simulink model "Simulasyon"  (R2022b)
settings: Solver=FixedStepDiscrete  StartTime=0.0  StopTime=0.05  FixedStep=1e-7  RelTol=1e-3
undefined symbols (not defined in the file): Ion, Lithium
libraries: spsSeriesRLCBranchLib x10, spsMosfetLib x8, spsPWMGenerator2LevelLib x5, spsThreePhaseVIMeasurementLib x4, spsThreePhaseSeriesRLCBranchLib x4, spsVoltageMeasurementLib x3, spsThreePhaseParallelRLCLoadLib x2, spsDCVoltageSourceLib x2, spsIGBTLib x2, spsThreePhaseBreakerLib x2, spsBatteryLib x1, spsBoostConverterLib x1
settings Model: Creator=ERKAM  LastModifiedBy=ERKAM
settings DataIOCC: ReturnWorkspaceOutputs=off

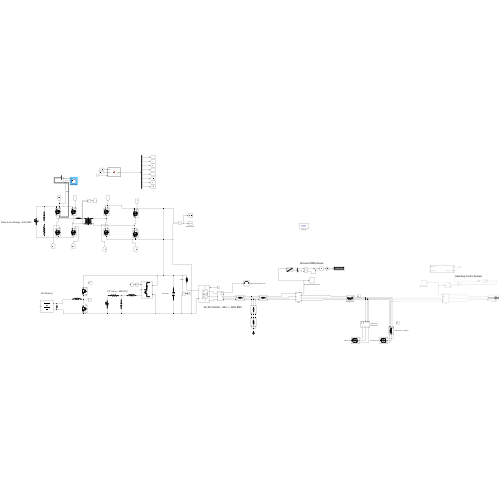
[thumbnail: Simulink's stored preview of the top-level diagram]
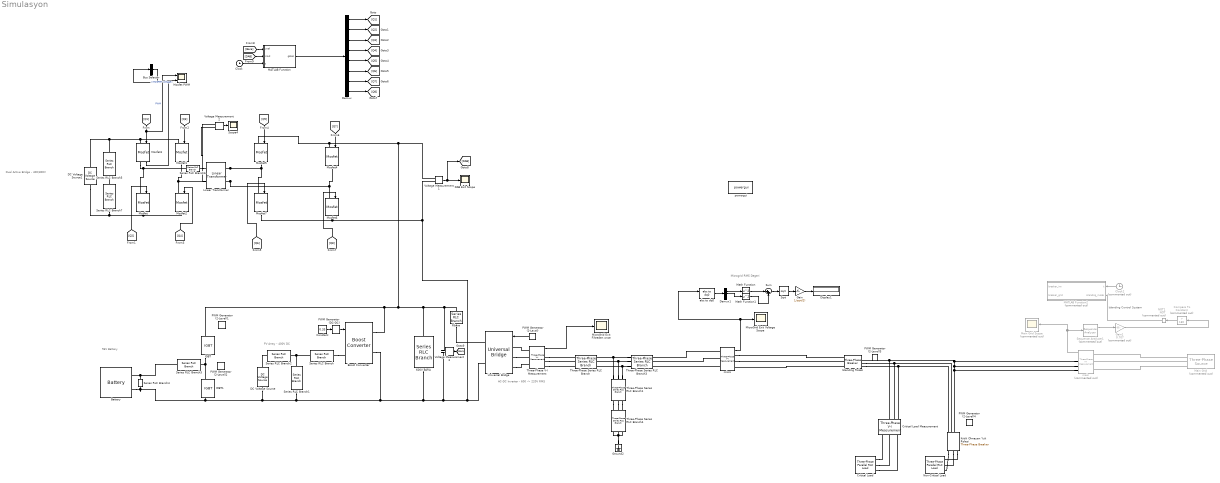
== system Simulasyon ==
  note: Islanding Control System
  note: AC-DC Inverter - 600 -> 220V RMS
  note: Dual Active Bridge - 400/800V
  note: PV Array - 400V DC
  note: 96V Battery
  note: Microgrid RMS Degeri
  600V BARA : spsSeriesRLCBranchLib/Series RLC Branch  LConnTagsString=__new0  RConnTagsString=__new0  BranchType=C  Resistance=1  Inductance=1e-3  SetiL0=off  InitialCurrent=0  Capacitance=100e-6  Setx0=on  InitialVoltage=600  Measurements=None
  Battery : spsBatteryLib/Battery  BatType=Lithium-Ion  ShowTempParam=off  ThermalPreset=no  ShowAgeParam=off  NomV=96  NomQ=100  SOC=100  Batt_Tr=30  PresetModel=on  MaxQ=100  MinV=72  FullV=111.7428  Dis_rate=43.4783  R=0.0096  Normal_OP=90.4348  expZone="[103.717      4.913043]"  current=[6.5 13 32.5]  Units=Time  Tci=20  NomT=20  T2=-30  MaxQ2=4.8  FullV2=7.1  Normal_OP2=5.655  expZone2="[6.58           1]"  Rca=0.6  ti=2000  Dp=0  Neq0=0  Tsim=1e6  Ta1=25  Qeol=5.4*0.9  Reol=0.013333*1.2  Char_age=[2.3478, 3]  Dis_age=[2.3478, 10]  N1=1500  N2=10500  N3=1000  N4=1400  Ta2=45  N5=950
  Boost Converter : spsBoostConverterLib/Boost Converter  ModelType=Switching devices  Ron=1e-3  Rs=1e6  Cs=inf  Vforward=[0,0]  Ron_Diode=1e-3  Rs_Diode=1e6  Cs_Diode=inf  Vf_Diode=1e-3  Rs_CurrentSource=inf  Ron_ACsource=1e-3
      settings: LibrarySourceBlock=sps_lib/Power Electronics/Boost Converter
  Bus Selector : BusSelector  OutputSignals=MOSFET voltage
  Clock : Clock
  Clock2 : Clock  Commented=on
  Compare To Constant : simulink/Logic and Bit Operations/Compare To Constant  Commented=on  relop=>  const=180  OutDataTypeStr=boolean
  Constant : Constant  Value=0.33  SampleTime=1e-7
  Critical Load : spsThreePhaseParallelRLCLoadLib/Three-Phase Parallel RLC Load  LConnTagsString=A|B|C  Configuration=Y (grounded)  NominalVoltage=220  Vabc=[1e3 1e3 1e3]  Vabcp=[1e3 1e3 1e3]  NominalFrequency=50  UnbalancedPower=off  ActivePower=1000  InductivePower=100  CapacitivePower=100  Pabc=[10e3 9e3 11e3]  QLabc=[100 90 110]  QCabc=[100 90 110]  Pabcp=[10e3 9e3 11e3]  QLabcp=[100 90 110]  QCabcp=[100 90 110]  Measurements=None  LoadType=constant Z
  Critical Load Measurement : spsThreePhaseVIMeasurementLib/Three-Phase V-I Measurement  VoltageMeasurement=phase-to-ground  SetLabelV=off  LabelV=Vabc  Vpu=off  VpuLL=off  CurrentMeasurement=yes  SetLabelI=off  LabelI=Iabc  Ipu=off  Pbase=100e6  Vbase=500e3  OutputType=Complex  PhasorSimulation=off  PSBequivalent=0
  DAB Exit Scope : Scope
  DC Voltage Source : spsDCVoltageSourceLib/DC Voltage Source  Amplitude=400  Measurements=None
  DC Voltage Source1 : spsDCVoltageSourceLib/DC Voltage Source  Amplitude=400  Measurements=Voltage
  Demux : Demux  Outputs=8
  Demux1 : Demux  Outputs=3
  Display1 : Display
  Gain : Gain  Gain=1/sqrt(2)
  Gain1 : Gain  Commented=on  Gain=0.707
  Ground2 : spsGroundLib/Ground  LConnTagsString=a
  IGBT : spsIGBTLib/IGBT  Ron=0.001  Lon=0  Vf=1  Tf=1e-6  Tt=2e-6  IC=0  Rs=1e5  Cs=inf  Measurements=on
  IGBT1 : spsIGBTLib/IGBT  Ron=0.001  Lon=0  Vf=1  Tf=1e-6  Tt=2e-6  IC=0  Rs=1e5  Cs=inf  Measurements=on
  Islanding Rolesi : spsThreePhaseBreakerLib/Three-Phase Breaker  InitialState=closed  SwitchA=on  SwitchB=on  SwitchC=on  SwitchTimes="[1/60  5/60]"  External=on  BreakerResistance=0.01  SnubberResistance=1e6  SnubberCapacitance=inf  Measurements=None
  Kritik Olmayan Yuk Rolesi : spsThreePhaseBreakerLib/Three-Phase Breaker  InitialState=closed  SwitchA=on  SwitchB=on  SwitchC=on  SwitchTimes="[1/60  5/60]"  External=on  BreakerResistance=0.01  SnubberResistance=1e6  SnubberCapacitance=inf  Measurements=None
  Linear Transformer : spsLinearTransformerLib/Linear Transformer  UNITS=SI  NominalPower=[10000 100000 ]  winding1=[400 0.1 0]  winding2=[400 0.1 0]  ThreeWindings=off  winding3=[3.15e+05 0.7938 0.084225]  RmLm=[1.0804e+06 2.55e-3]  Measurements=None  DataType=on
  MATLAB Function : MATLAB Function  TreatAsAtomicUnit=on  SystemSampleTime=1e-7
  MATLAB Function2 : MATLAB Function  Commented=on  TreatAsAtomicUnit=on
  Main Grid : spsThreePhaseSourceLib/Three-Phase Source  Commented=on  InternalConnection=Yg  VoltagePhases=off  Voltage=220  PhaseAngle=0  Voltage_phases=[25e3 25e3 25e3]/sqrt(3)  PhaseAngles_phases=[0 -120 +120]  Frequency=50  NonIdealSource=off  SpecifyImpedance=off  Resistance=0.8929  Inductance=16.58e-3  ShortCircuitLevel=100e6  BaseVoltage=25e3  XRratio=7  BusType=swing  Pref=300  Qref=0  Prefabc=[10e3, 10e3, 10e3]  Qrefabc=[0, 0, 0]  Qmin=-inf  Qmax=inf
  Main Grid Scope : Scope  Commented=on
  Math Function : Math  Operator=square
  Math Function1 : Math  Operator=square
  MicroGrid Exit Filtreden once : Scope
  MicroGrid Exit Voltage Scope : Scope
  Mosfet{,1..2,4..7} (7 alike) : spsMosfetLib/Mosfet  Ron=0.1  Lon=0  Rd=0.01  Vfd=0  IC=0  Rs=1e5  Cs=inf  Measurements=off
  Mosfet PWM : Scope  NumInputPorts=2
  Mosfet3 : spsMosfetLib/Mosfet  Ron=0.1  Lon=0  Rd=0.01  Vfd=0  IC=0  Rs=1e5  Cs=inf  Measurements=on
  NOT1 : Logic  Commented=on  Operator=NOT  IconShape=distinctive  AllPortsSameDT=off  OutDataTypeStr=boolean
  Non-Critical Load : spsThreePhaseParallelRLCLoadLib/Three-Phase Parallel RLC Load  LConnTagsString=A|B|C  Configuration=Y (grounded)  NominalVoltage=220  Vabc=[1e3 1e3 1e3]  Vabcp=[1e3 1e3 1e3]  NominalFrequency=50  UnbalancedPower=off  ActivePower=1000  InductivePower=100  CapacitivePower=100  Pabc=[10e3 9e3 11e3]  QLabc=[100 90 110]  QCabc=[100 90 110]  Pabcp=[10e3 9e3 11e3]  QLabcp=[100 90 110]  QCabcp=[100 90 110]  Measurements=None  LoadType=constant Z
  PWM Generator (2-Level) : spsPWMGenerator2LevelLib/PWM Generator (2-Level)  ModulatorType=Three-phase bridge (6 pulses)  ModulatorMode=Unsynchronized  Fc=100000  Pc=0  nF=27  MinMax="[ -1  1 ]"  SamplingTechnique=Natural  ModulatingSignals=on  m=0.98  Freq=50  Phase=90  Ts=1e-7  ShowCarrierOutport=off
  PWM Generator (2-Level)1 : spsPWMGenerator2LevelLib/PWM Generator (2-Level)  ModulatorType=Three-phase bridge (6 pulses)  ModulatorMode=Unsynchronized  Fc=100000  Pc=0  nF=27  MinMax="[ -1  1 ]"  SamplingTechnique=Natural  ModulatingSignals=on  m=0.98  Freq=50  Phase=90  Ts=1e-7  ShowCarrierOutport=off
  PWM Generator (2-Level)2 : spsPWMGenerator2LevelLib/PWM Generator (2-Level)  ModulatorType=Three-phase bridge (6 pulses)  ModulatorMode=Unsynchronized  Fc=100000  Pc=0  nF=27  MinMax="[ -1  1 ]"  SamplingTechnique=Natural  ModulatingSignals=on  m=0.98  Freq=50  Phase=90  Ts=1e-7  ShowCarrierOutport=off
  PWM Generator (2-Level)3 : spsPWMGenerator2LevelLib/PWM Generator (2-Level)  ModulatorType=Three-phase bridge (6 pulses)  ModulatorMode=Unsynchronized  Fc=100000  Pc=0  nF=27  MinMax="[ -1  1 ]"  SamplingTechnique=Natural  ModulatingSignals=on  m=0  Freq=50  Phase=90  Ts=1e-7  ShowCarrierOutport=off
  PWM Generator (2-Level)4 : spsPWMGenerator2LevelLib/PWM Generator (2-Level)  ModulatorType=Three-phase bridge (6 pulses)  ModulatorMode=Unsynchronized  Fc=100000  Pc=0  nF=27  MinMax="[ -1  1 ]"  SamplingTechnique=Natural  ModulatingSignals=on  m=0  Freq=50  Phase=90  Ts=1e-7  ShowCarrierOutport=off
  PWM Generator (DC-DC) : spsPWMGeneratorDCDCLib/PWM Generator (DC-DC)  Fsw=100000  Ts=1e-7
  Rbara : spsSeriesRLCBranchLib/Series RLC Branch  LConnTagsString=__new0  RConnTagsString=__new0  BranchType=R  Resistance=10e-3  Inductance=1e-3  SetiL0=off  InitialCurrent=0  Capacitance=100e-6  Setx0=on  InitialVoltage=600  Measurements=None
  Scope4 : Scope
  Sequence Analyzer1 : spsSequenceAnalyzerLib/Sequence Analyzer  Commented=on  Freq=50  n=1  seq=Positive  InInit=[1, 0]  Ts=1e-7
      settings: LibrarySourceBlock=sps_lib/Sensors and Measurements/Sequence Analyzer
  Series RLC Branch : spsSeriesRLCBranchLib/Series RLC Branch  LConnTagsString=__new0  RConnTagsString=__new0  BranchType=L  Resistance=1  Inductance=5e-3  SetiL0=off  InitialCurrent=0  Capacitance=1e-6  Setx0=off  InitialVoltage=0  Measurements=None
  Series RLC Branch1 : spsSeriesRLCBranchLib/Series RLC Branch  LConnTagsString=__new0  RConnTagsString=__new0  BranchType=C  Resistance=1  Inductance=1e-3  SetiL0=off  InitialCurrent=0  Capacitance=45e-6  Setx0=off  InitialVoltage=0  Measurements=None
  Series RLC Branch2 : spsSeriesRLCBranchLib/Series RLC Branch  LConnTagsString=__new0  RConnTagsString=__new0  BranchType=R  Resistance=1  Inductance=5e-3  SetiL0=off  InitialCurrent=0  Capacitance=1e-6  Setx0=off  InitialVoltage=0  Measurements=None
  Series RLC Branch3 : spsSeriesRLCBranchLib/Series RLC Branch  LConnTagsString=__new0  RConnTagsString=__new0  BranchType=L  Resistance=1  Inductance=2e-3  SetiL0=off  InitialCurrent=0  Capacitance=1e-6  Setx0=off  InitialVoltage=0  Measurements=None
  Series RLC Branch4 : spsSeriesRLCBranchLib/Series RLC Branch  LConnTagsString=__new0  RConnTagsString=__new0  BranchType=C  Resistance=1  Inductance=2e-3  SetiL0=off  InitialCurrent=0  Capacitance=5.066e-6  Setx0=off  InitialVoltage=0  Measurements=None
  Series RLC Branch5 : spsSeriesRLCBranchLib/Series RLC Branch  LConnTagsString=__new0  RConnTagsString=__new0  BranchType=C  Resistance=1000  Inductance=1e-3  SetiL0=off  InitialCurrent=0  Capacitance=470e-6  Setx0=off  InitialVoltage=0  Measurements=None
  Series RLC Branch6 : spsSeriesRLCBranchLib/Series RLC Branch  LConnTagsString=__new0  RConnTagsString=__new0  BranchType=L  Resistance=1000  Inductance=20e-6  SetiL0=off  InitialCurrent=0  Capacitance=470e-6  Setx0=off  InitialVoltage=0  Measurements=None
  Series RLC Branch7 : spsSeriesRLCBranchLib/Series RLC Branch  LConnTagsString=__new0  RConnTagsString=__new0  BranchType=R  Resistance=50  Inductance=1e-3  SetiL0=off  InitialCurrent=0  Capacitance=470e-6  Setx0=off  InitialVoltage=0  Measurements=None
  Sqrt : Sqrt
  Sum : Sum  Inputs=|++
  Three-Phase Series RLC Branch : spsThreePhaseSeriesRLCBranchLib/Three-Phase Series RLC Branch  LConnTagsString=A|B|C  RConnTagsString=A|B|C  BranchType=L  Resistance=1  Inductance=2e-3  Capacitance=1e-6  Measurements=None
  Three-Phase Series RLC Branch1 : spsThreePhaseSeriesRLCBranchLib/Three-Phase Series RLC Branch  LConnTagsString=A|B|C  RConnTagsString=A|B|C  BranchType=C  Resistance=1  Inductance=1e-3  Capacitance=25e-6  Measurements=None
  Three-Phase Series RLC Branch3 : spsThreePhaseSeriesRLCBranchLib/Three-Phase Series RLC Branch  LConnTagsString=A|B|C  RConnTagsString=A|B|C  BranchType=L  Resistance=1  Inductance=2e-3  Capacitance=1e-6  Measurements=None
  Three-Phase Series RLC Branch4 : spsThreePhaseSeriesRLCBranchLib/Three-Phase Series RLC Branch  LConnTagsString=A|B|C  RConnTagsString=A|B|C  BranchType=R  Resistance=42  Inductance=2e-3  Capacitance=1e-6  Measurements=None
  Three-Phase V-I Measurement : spsThreePhaseVIMeasurementLib/Three-Phase V-I Measurement  VoltageMeasurement=phase-to-phase  SetLabelV=off  LabelV=Vabc  Vpu=off  VpuLL=off  CurrentMeasurement=yes  SetLabelI=off  LabelI=Iabc  Ipu=off  Pbase=100e6  Vbase=500e3  OutputType=Complex  PhasorSimulation=off  PSBequivalent=0
  Universal Bridge : spsUniversalBridgeLib/Universal Bridge  Arms=3  SnubberResistance=1e5  SnubberCapacitance=100e-6  Device=MOSFET / Diodes  Ron=1e-3  Lon=0  ForwardVoltages="[  0  0  ]"  ForwardVoltage=0  GTOparameters=[ 10e-6 , 20e-6 ]  IGBTparameters=[ 1e-6 , 2e-6 ]  Measurements=None  Measurements_2=None  converterType=Rectifier
  Voltage Measurement1 : spsVoltageMeasurementLib/Voltage Measurement  PhasorSimulation=off  OutputType=Complex  PSBequivalent=0
  Voltage Measurement2 : spsVoltageMeasurementLib/Voltage Measurement  PhasorSimulation=off  OutputType=Complex  PSBequivalent=0
  Voltage Measurement3 : spsVoltageMeasurementLib/Voltage Measurement  PhasorSimulation=off  OutputType=Complex  PSBequivalent=0
  abc to dq0 : spsabctodq0Lib/abc to dq0  Alignment=90 degrees behind phase A axis
  main : spsThreePhaseVIMeasurementLib/Three-Phase V-I Measurement  Commented=on  VoltageMeasurement=phase-to-phase  SetLabelV=off  LabelV=Vabc  Vpu=off  VpuLL=off  CurrentMeasurement=yes  SetLabelI=off  LabelI=Iabc  Ipu=off  Pbase=100e6  Vbase=500e3  OutputType=Complex  PhasorSimulation=off  PSBequivalent=0
  micro : spsThreePhaseVIMeasurementLib/Three-Phase V-I Measurement  VoltageMeasurement=phase-to-phase  SetLabelV=off  LabelV=Vabc  Vpu=off  VpuLL=off  CurrentMeasurement=no  SetLabelI=off  LabelI=Iabc  Ipu=off  Pbase=100e6  Vbase=500e3  OutputType=Complex  PhasorSimulation=off  PSBequivalent=0
  powergui : spspowerguiLib/powergui  Priority=1  SimulationMode=Discrete  SampleTime=1e-7  frequency=60  Iterations=50  frequencyindice=0  Pbase=100e6  ErrMax=1e-4  UnitsV=kV  UnitsW=MW  buscounter=0  FunctionMessages=off  echomessages=off  EnableUseOfTLC=off  CurrentSourceSwitches=off  DisableSnubberDevices=off  DisableRonSwitches=off  DisableVfSwitches=off  DisplayEquations=off  AutomaticDiscreteSolvers=off  SolverType=Tustin/Backward Euler (TBE)  Interpol=off  ExternalGateDelay=off  methode=off  Ts=100  x0status=blocks  SPID=on  SwTol=0  HookPort=off  NonlinearTolerance=1e-4  nMaxIteration=100  ContinueOnMaxIteration=off  RestoreLinks=warning  ResistiveCurrentMeasurement=off  Frange=[0:2:500]  Ylog=off  Xlog=on  ShowGrid=off  save=off  variable=ZData  structure=0  ZoomFFT=off  StartTime=0.0  cycles=1  DisplayStyle=1  fundamental=60  FreqAxis=off  MaxFrequency=1000  frequencyindicesteady=1  RmsSteady=1  display=off
  wires:
  Gain1/1 -> Compare To Constant/1
  Compare To Constant/1 -> NOT1/1
  micro/1 -> abc to dq0/1, MicroGrid Exit Voltage Scope/1
  Sequence Analyzer1/1 -> Gain1/1
  main/1 -> Main Grid Scope/1, Sequence Analyzer1/1
  PWM Generator (DC-DC)/1 -> Boost Converter/1
  Constant/1 -> PWM Generator (DC-DC)/1
  Voltage Measurement1/1 -> [DAB], DAB Exit Scope/1
  Voltage Measurement2/1 -> Scope4/1
  Clock/1 -> MATLAB Function/3(t)
  Demux/1 -> [Q1]
  [Q1] -> Mosfet PWM/1, Mosfet3/1  "PWM"
  [Q4] -> Mosfet2/1
  [Q8] -> Mosfet6/1
  [Q5] -> Mosfet5/1
  Demux/2 -> [Q2]
  Demux/3 -> [Q3]
  Demux/4 -> [Q4]
  Demux/5 -> [Q5]
  Demux/6 -> [Q6]
  Demux/7 -> [Q7]
  Demux/8 -> [Q8]
  MATLAB Function/1(gates) -> Demux/1
  [Q2] -> Mosfet/1
  [Q3] -> Mosfet1/1
  [Q7] -> Mosfet4/1
  [Q6] -> Mosfet7/1
  Voltage Measurement3/1 -> [Bara]
  PWM Generator (2-Level)/1 -> Universal Bridge/1
  [Bara] -> MATLAB Function/1(Vref)
  Clock2/1 -> MATLAB Function2/1(t)
  NOT1/1 -> MATLAB Function2/2(islanding_mode)
  Three-Phase V-I Measurement/1 -> MicroGrid Exit Filtreden once/1
  [DAB] -> MATLAB Function/2(Vout)
  abc to dq0/1 -> Demux1/1
  Demux1/1 -> Math Function/1
  Demux1/2 -> Math Function1/1
  Math Function/1 -> Sum/1
  Math Function1/1 -> Sum/2
  Sum/1 -> Sqrt/1
  Sqrt/1 -> Gain/1
  Gain/1 -> Display1/1
  Mosfet3/1 -> Bus Selector/1
  Bus Selector/1 -> Mosfet PWM/2  "<MOSFET voltage>"
  connections:
  Voltage Measurement1/LConn1 -- Mosfet5/LConn1 -- Mosfet4/LConn1 -- IGBT/LConn1 -- Boost Converter/RConn1 -- Rbara/LConn1 -- Voltage Measurement3/LConn1 -- 600V BARA/LConn1
  Three-Phase V-I Measurement/LConn1 -- Universal Bridge/LConn1
  Universal Bridge/LConn2 -- Three-Phase V-I Measurement/LConn2
  Universal Bridge/LConn3 -- Three-Phase V-I Measurement/LConn3
  Three-Phase Series RLC Branch3/LConn1 -- Three-Phase Series RLC Branch1/LConn1 -- Three-Phase Series RLC Branch/RConn1
  Three-Phase Series RLC Branch3/LConn2 -- Three-Phase Series RLC Branch1/LConn2 -- Three-Phase Series RLC Branch/RConn2
  Three-Phase Series RLC Branch3/LConn3 -- Three-Phase Series RLC Branch1/LConn3 -- Three-Phase Series RLC Branch/RConn3
  Kritik Olmayan Yuk Rolesi/LConn3 -- Islanding Rolesi/LConn3 -- Critical Load Measurement/RConn3
  Kritik Olmayan Yuk Rolesi/LConn2 -- Critical Load Measurement/RConn2 -- Islanding Rolesi/LConn2
  Critical Load Measurement/RConn1 -- main/RConn1 -- main/RConn2 -- main/RConn3 -- Kritik Olmayan Yuk Rolesi/LConn1 -- Islanding Rolesi/LConn1
  Three-Phase V-I Measurement/RConn1 -- Three-Phase Series RLC Branch/LConn1
  Three-Phase V-I Measurement/RConn2 -- Three-Phase Series RLC Branch/LConn2
  Three-Phase V-I Measurement/RConn3 -- Three-Phase Series RLC Branch/LConn3
  Three-Phase Series RLC Branch1/RConn1 -- Three-Phase Series RLC Branch4/LConn1
  Three-Phase Series RLC Branch1/RConn2 -- Three-Phase Series RLC Branch4/LConn2
  Three-Phase Series RLC Branch1/RConn3 -- Three-Phase Series RLC Branch4/LConn3
  Main Grid/RConn1 -- main/LConn1
  Main Grid/RConn2 -- main/LConn2
  Main Grid/RConn3 -- main/LConn3
  Series RLC Branch1/LConn1 -- Series RLC Branch2/RConn1 -- Series RLC Branch/LConn1
  Series RLC Branch/RConn1 -- Boost Converter/LConn1
  Series RLC Branch2/LConn1 -- DC Voltage Source/RConn1
  Three-Phase Series RLC Branch4/RConn2 -- Three-Phase Series RLC Branch4/RConn3 -- Ground2/LConn1 -- Three-Phase Series RLC Branch4/RConn1
  Voltage Measurement1/LConn2 -- Universal Bridge/RConn2 -- Voltage Measurement3/LConn2 -- Series RLC Branch4/RConn1 -- Battery/LConn2 -- IGBT1/RConn1 -- DC Voltage Source/LConn1 -- Series RLC Branch1/RConn1 -- Boost Converter/RConn2 -- 600V BARA/RConn1 -- Mosfet7/RConn1 -- Mosfet6/RConn1
  Mosfet3/RConn1 -- Series RLC Branch6/LConn1 -- Mosfet/LConn1
  Mosfet1/RConn1 -- Linear Transformer/LConn2 -- Mosfet2/LConn1
  Mosfet3/LConn1 -- Series RLC Branch5/LConn1 -- DC Voltage Source1/RConn1 -- Mosfet1/LConn1
  Mosfet/RConn1 -- Series RLC Branch7/RConn1 -- DC Voltage Source1/LConn1 -- Mosfet2/RConn1
  Mosfet5/RConn1 -- Voltage Measurement2/LConn1 -- Linear Transformer/RConn1 -- Mosfet7/LConn1
  Mosfet6/LConn1 -- Voltage Measurement2/LConn2 -- Linear Transformer/RConn2 -- Mosfet4/RConn1
  Series RLC Branch6/RConn1 -- Linear Transformer/LConn1
  Series RLC Branch7/LConn1 -- Series RLC Branch5/RConn1
  IGBT/RConn1 -- IGBT1/LConn1 -- Series RLC Branch3/RConn1
  Series RLC Branch3/LConn1 -- Series RLC Branch4/LConn1 -- Battery/LConn1
  micro/RConn1 -- Islanding Rolesi/RConn1
  micro/RConn2 -- Islanding Rolesi/RConn2
  Islanding Rolesi/RConn3 -- micro/RConn3
  Critical Load/LConn1 -- Critical Load Measurement/LConn1
  Critical Load/LConn2 -- Critical Load Measurement/LConn2
  Critical Load/LConn3 -- Critical Load Measurement/LConn3
  Kritik Olmayan Yuk Rolesi/RConn1 -- Non-Critical Load/LConn1
  Kritik Olmayan Yuk Rolesi/RConn2 -- Non-Critical Load/LConn2
  Kritik Olmayan Yuk Rolesi/RConn3 -- Non-Critical Load/LConn3
  micro/LConn1 -- Three-Phase Series RLC Branch3/RConn1
  micro/LConn2 -- Three-Phase Series RLC Branch3/RConn2
  micro/LConn3 -- Three-Phase Series RLC Branch3/RConn3
  Rbara/RConn1 -- Universal Bridge/RConn1

== matlab function Simulasyon/MATLAB Function2 ==
  data: t input; breaker_inv output; islanding_mode input; breaker_grid output
function [breaker_inv, breaker_grid] = grid_control(t, islanding_mode)

if islanding_mode == 1
    % Ada modu: şebeke kesildi, invertör besliyor
    breaker_inv  = 1;
    breaker_grid = 0;
else
    % Normal mod: şebeke var, invertör senkronize oluyor
    breaker_inv  = 0;  % veya 1, paralel bağlantı için
    breaker_grid = 1;
end

== matlab function Simulasyon/MATLAB Function ==
  data: Vref input; gates output; Vout input; t input
function gates = fcn(Vref, Vout, t)
    fsw = 100000;
    T = 1/fsw;
    Ts = 1e-7;

    persistent error_int phi_prev
    if isempty(error_int)
        error_int = 0;
    end
    if isempty(phi_prev)
        phi_prev = 0.1;
    end

    Kp = 0.001;
    Ki = 0.005;

    error = Vref - Vout;

    % Phi hesapla
    phi_raw = (Kp * error) + (Ki * error_int);

    % Sınır kontrolü
    phi_raw = max(0, min(0.25, phi_raw));

    % Rate limiter — ani zıplamayı önle
    max_delta = 0.005;
    phi_raw = max(phi_prev - max_delta, min(phi_prev + max_delta, phi_raw));
    phi_prev = phi_raw;

    % Anti-windup — sadece sınır içindeyse integral biriktir
    if phi_raw > 0 && phi_raw < 0.25
        error_int = error_int + (error * Ts);
        error_int = max(-50, min(50, error_int));
    end

    shift_ratio = phi_raw;
    phi_time = shift_ratio * T;

    % PWM üretimi
    t_mod = mod(t, T);

    g1 = (t_mod < T/2);
    g2 = ~g1;
    g3 = (t_mod >= T/2);
    g4 = ~g3;

    ts = mod(t - phi_time, T);
    g5 = (ts < T/2);
    g6 = ~g5;
    g7 = (ts >= T/2);
    g8 = ~g7;

    gates = [g1 g2 g3 g4 g5 g6 g7 g8];
end
